simulink model "MARQUEZ_NO2_SIMULINK"  (R2023b)
settings: Solver=VariableStepAuto  StartTime=0.0  StopTime=20.0  RelTol=1e-3
values from neighbouring files (symbols this model uses):
  E_den = [M B k]    [Marquez_No2.m]
  E_num = [1]    [Marquez_No2.m]
settings Model: Creator=Princess  LastModifiedBy=Princess

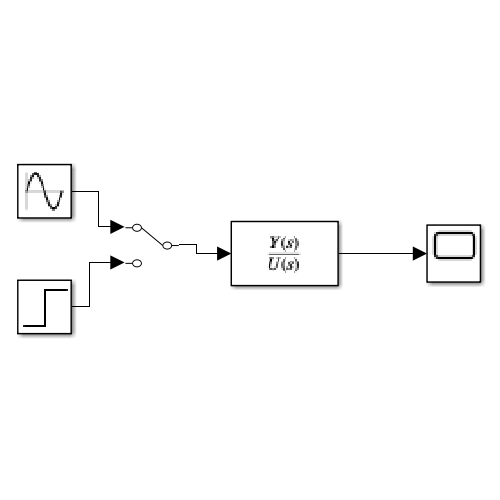
[thumbnail: Simulink's stored preview of the top-level diagram]
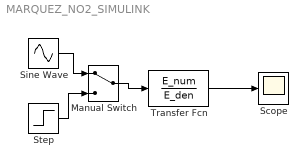
== system MARQUEZ_NO2_SIMULINK ==
  Manual Switch : ManualSwitch
  Scope : Scope
  Sine Wave : Sin  Amplitude=0  SampleTime=0
  Step : Step  SampleTime=0
  Transfer Fcn : TransferFcn  Numerator=E_num  Denominator=E_den
  wires:
  Manual Switch/1 -> Transfer Fcn/1
  Step/1 -> Manual Switch/2
  Sine Wave/1 -> Manual Switch/1
  Transfer Fcn/1 -> Scope/1
